simulink model "LR_Traject_Sim"  (R2017b)
settings: Solver=ode4  StartTime=0  StopTime=100  FixedStep=0.05  RelTol=1e-7
model workspace (MAT data in the model file):
  Object = Simulink.LookupTable
  Object.Table = Simulink.lookuptable.Table
  Object.Table.Dimensions = [0 0]
  Object.Table.DataType = 'auto'
  Object.Table.FieldName = 'Table'
  Object.Breakpoints = Simulink.lookuptable.Breakpoint
  Object.Breakpoints.TunableSizeName = 'N1'
  Object.Breakpoints.Dimensions = [0 0]
  Object.Breakpoints.DataType = 'auto'
  Object.Breakpoints.FieldName = 'BP1'
  Object.SupportTunableSize = 0
  Object.StructTypeInfo = Simulink.lookuptable.StructTypeInfo
  Object.StructTypeInfo.DataScope = 'Auto'
values from neighbouring files (symbols this model uses):
  Vull = 0.15    [TestBlowdownModel.m]    (also in runsim.m)
undefined symbols (not defined in the file or in its folder): CEAinterp, Conditions, Eng, Prop, Roc
libraries: simulink x1
settings Model: Creator=adamb  LastModifiedBy=Thomas
settings SolverCC: ZeroCrossAlgorithm=Adaptive
settings DataIOCC: SaveFormat=StructureWithTime
settings OptimizationCC: LifeSpan=inf
settings DebuggingCC: AlgebraicLoopMsg=none  ArtificialAlgebraicLoopMsg=none  SFExecutionAtInitializationDiag=none
settings HardwareCC: ProdBitPerSizeT=32  ProdBitPerPtrDiffT=32  ProdWordSize=32  ProdHWDeviceType=Specified
settings CodeAppCC: StateflowObjectComments=on
settings SimscapeCC: SimscapeNormalizeSystem=off
settings ConfigurationSet: Description=SimMechanics 2G

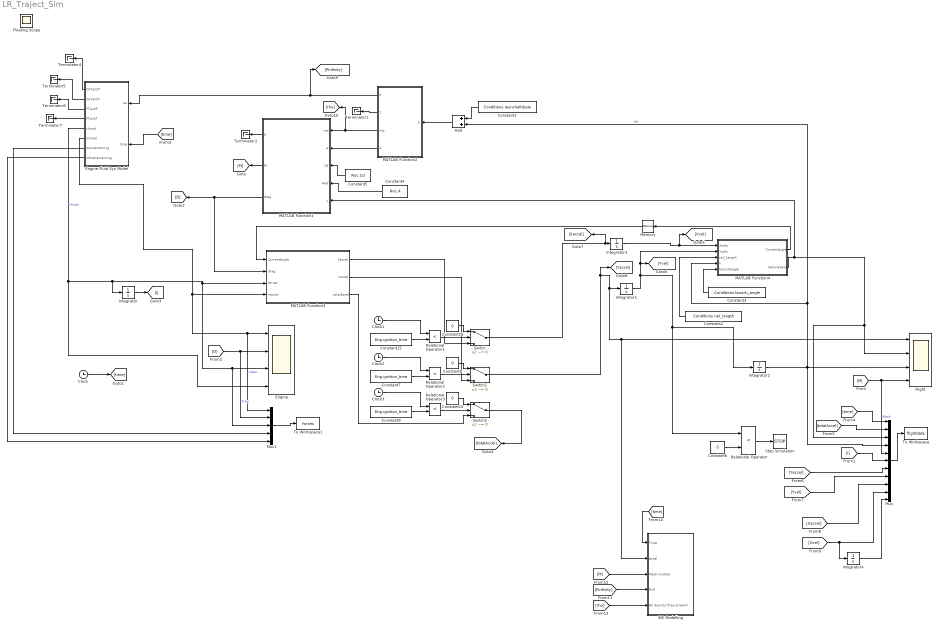
== system LR_Traject_Sim ==
  Add : Sum
  Clock{,1..3} (4 alike) : Clock
  Constant1 : Constant  Value=Conditions.launchaltitude
  Constant10 : Constant  Value=0
  Constant15 : Constant  Value=Eng.ignition_time
  Constant16 : Constant  Value=0
  Constant2 : Constant  Value=Conditions.rail_length
  Constant3 : Constant  Value=Conditions.launch_angle
  Constant4 : Constant  Value=Roc.A
  Constant5 : Constant  Value=Roc.Cd  VectorParams1D=off
  Constant6 : Constant  Value=-5
  Constant7 : Constant  Value=Eng.ignition_time
  Constant8 : Constant  Value=0
  Constant9 : Constant  Value=Eng.ignition_time
  Engine : Scope  NumInputPorts=4
  Engine Fluid Sys Model : Subsystem
  Flight : Scope  NumInputPorts=4
  INS Modelling : Subsystem
  Integrator{,1..4} (5 alike) : Integrator
  MATLAB Function1 : MATLAB Function  TreatAsAtomicUnit=on
  MATLAB Function2 : MATLAB Function  TreatAsAtomicUnit=on
  MATLAB Function3 : MATLAB Function  TreatAsAtomicUnit=on
  MATLAB Function4 : MATLAB Function  TreatAsAtomicUnit=on
  Memory : Memory
  Mux : Mux  Inputs=11
  Mux1 : Mux  Inputs=5
  Relational Operator : RelationalOperator  Operator=<  OutDataTypeStr=boolean  RndMeth=Nearest
  Relational Operator1 : RelationalOperator  Operator=<  OutDataTypeStr=boolean  RndMeth=Simplest
  Relational Operator2 : RelationalOperator  Operator=<  OutDataTypeStr=boolean  RndMeth=Simplest
  Relational Operator3 : RelationalOperator  Operator=<  OutDataTypeStr=boolean  RndMeth=Simplest
  Stop Simulation : Stop
  Switch : Switch  Criteria=u2 ~= 0
  Switch1 : Switch  Criteria=u2 ~= 0
  Switch2 : Switch  Criteria=u2 ~= 0
  Terminator{1..2,4..7} (6 alike) : Terminator
  To Workspace : ToWorkspace  VariableName=flightdata  SampleTime=-1
  To Workspace1 : ToWorkspace  VariableName=forces  SampleTime=-1
  Floating Scope : Scope
  wires:
  Engine Fluid Sys Model/6(mtotal) -> Mux1/1, Engine/1, MATLAB Function3/4(mtotal)  "mass"
  Engine Fluid Sys Model/5(thrust) -> Integrator/1, Mux1/3, Engine/3, MATLAB Function3/3(thrust), Engine/4  "thrust"
  Integrator1/1 -> Relational Operator/1, Integrator2/1, [Yvel], MATLAB Function4/2(Yvelo)
  Integrator2/1 -> Add/2, MATLAB Function4/4(h), Flight/3, Mux/4  "alt"
  Constant4/1 -> MATLAB Function1/4(Aref)
  Constant5/1 -> MATLAB Function1/3(Cd)
  MATLAB Function1/2(M) -> [M]
  [M] -> Mux/5, Flight/4  "Mach"
  MATLAB Function1/3(drag) -> [D], MATLAB Function3/2(drag)
  Relational Operator/1 -> Stop Simulation/1
  Constant6/1 -> Relational Operator/2
  MATLAB Function2/4(a) -> MATLAB Function1/2(a)
  MATLAB Function2/3(rho) -> [rho], MATLAB Function1/1(rho)
  Mux/1 -> To Workspace/1
  MATLAB Function2/2(T) -> Terminator1/1
  [D] -> Mux1/2, Engine/2  "drag"
  Mux1/1 -> To Workspace1/1
  MATLAB Function1/1(q) -> Terminator2/1
  MATLAB Function2/1(P) -> [Pinfinity], Engine Fluid Sys Model/1(pa)
  Clock/1 -> [time]
  [time] -> Engine Fluid Sys Model/2(time)
  [time] -> Mux/1
  Engine Fluid Sys Model/7(moxremaining) -> Mux1/4
  Engine Fluid Sys Model/8(mfuelremaining) -> Mux1/5
  Switch1/1 -> [Yaccel], INS Modelling/2(Accel), Flight/1, Integrator1/1
  Integrator3/1 -> [Xvel], MATLAB Function4/1(Xvelo)
  MATLAB Function4/2(VehicleVelo) -> MATLAB Function1/5(v), Flight/2, Mux/3
  Integrator/1 -> [I]
  [I] -> Mux/6
  Add/1 -> MATLAB Function2/1(h)
  Constant1/1 -> Add/1
  MATLAB Function4/1(CurrentAngle) -> Memory/1
  Engine Fluid Sys Model/1(OxTankP) -> Terminator4/1
  Engine Fluid Sys Model/2(OxTankT) -> Terminator5/1
  Engine Fluid Sys Model/3(FTankP) -> Terminator6/1
  Engine Fluid Sys Model/4(FTankT) -> Terminator7/1
  Constant2/1 -> MATLAB Function4/3(rail_length)
  Constant3/1 -> MATLAB Function4/5(launchangle)
  Memory/1 -> MATLAB Function3/1(CurrentAngle)
  [totalAccel] -> Mux/2
  [Xaccel] -> Mux/9
  [Xvel] -> Integrator4/1, Mux/10
  [Yvel] -> Mux/8
  [Yaccel] -> Mux/7
  Integrator4/1 -> Mux/11
  [time] -> INS Modelling/1(Time)
  [Pinfinity] -> INS Modelling/4(Pinf)
  [M] -> INS Modelling/3(Mach number)
  [rho] -> INS Modelling/5(Air density (free stream))
  Switch/1 -> Integrator3/1, [Xaccel]
  Clock1/1 -> Relational Operator1/1
  Relational Operator1/1 -> Switch/2
  Constant16/1 -> Switch/1
  Constant15/1 -> Relational Operator1/2
  Clock2/1 -> Relational Operator2/1
  Relational Operator2/1 -> Switch1/2
  Constant8/1 -> Switch1/1
  Constant7/1 -> Relational Operator2/2
  Clock3/1 -> Relational Operator3/1
  Relational Operator3/1 -> Switch2/2
  Constant10/1 -> Switch2/1
  Constant9/1 -> Relational Operator3/2
  MATLAB Function3/1(Xaccel) -> Switch/3
  MATLAB Function3/2(Yaccel) -> Switch1/3
  Switch2/1 -> [totalAccel]
  MATLAB Function3/3(totalAccel) -> Switch2/3

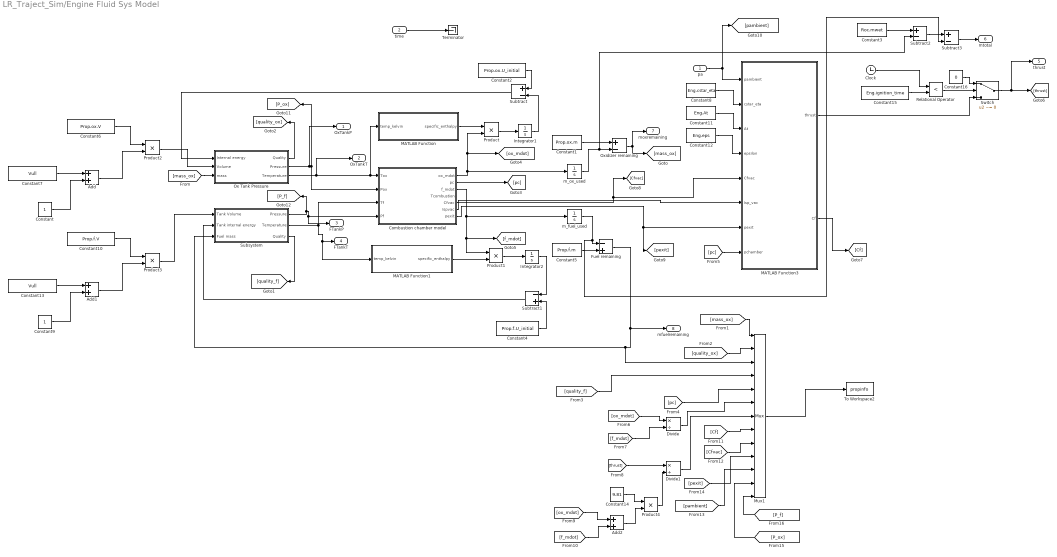
== system LR_Traject_Sim/Engine Fluid Sys Model ==
  pa : Inport
  time : Inport  Port=2
  Add : Sum
  Add1 : Sum
  Add2 : Sum
  Clock : Clock
  Combustion chamber model : Subsystem  TreatAsAtomicUnit=on
  Constant : Constant
  Constant1 : Constant  Value=Prop.ox.m
  Constant10 : Constant  Value=Prop.f.V
  Constant11 : Constant  Value=Eng.At
  Constant12 : Constant  Value=Eng.eps
  Constant13 : Constant  Value=Vull
  Constant14 : Constant  Value=9.81
  Constant15 : Constant  Value=Eng.ignition_time
  Constant16 : Constant  Value=0
  Constant2 : Constant  Value=Prop.ox.U_initial
  Constant3 : Constant  Value=Roc.mwet
  Constant4 : Constant  Value=Prop.f.U_initial
  Constant5 : Constant  Value=Prop.f.m
  Constant6 : Constant  Value=Prop.ox.V
  Constant7 : Constant  Value=Vull
  Constant8 : Constant  Value=Eng.cstar_eta
  Constant9 : Constant
  Divide : Product  Inputs=*/
  Divide1 : Product  Inputs=*/
  Fuel remaining : Sum  Inputs=-+
  Integrator1 : Integrator
  Integrator2 : Integrator
  MATLAB Function : MATLAB Function  TreatAsAtomicUnit=on
  MATLAB Function1 : MATLAB Function  TreatAsAtomicUnit=on
  MATLAB Function3 : MATLAB Function  TreatAsAtomicUnit=on
  Mux1 : Mux  Inputs=13
  Ox Tank Pressure : Subsystem  Variant=on  VariantControl=Variant1
  Oxidizer remaining : Sum  Inputs=+-
  Product{,1..4} (5 alike) : Product
  Relational Operator : RelationalOperator  Operator=<  OutDataTypeStr=boolean  RndMeth=Simplest
  Subsystem : Subsystem
  Subtract : Sum  Inputs=+-
  Subtract1 : Sum  Inputs=-+
  Subtract2 : Sum  Inputs=+-
  Subtract3 : Sum  Inputs=+-
  Switch : Switch  Criteria=u2 ~= 0
  Terminator : Terminator
  To Workspace2 : ToWorkspace  VariableName=propinfo  SampleTime=-1
  m_fuel_used : Integrator
  m_ox_used : Integrator
  OxTankP : Outport
  OxTankT : Outport  Port=2
  FTankP : Outport  Port=3
  FTankT : Outport  Port=4
  thrust : Outport  Port=5
  mtotal : Outport  Port=6
  moxremaining : Outport  Port=7
  mfuelremaining : Outport  Port=8
  wires:
  Constant11/1 -> MATLAB Function3/3(At)
  Constant12/1 -> MATLAB Function3/4(epsilon)
  Constant8/1 -> MATLAB Function3/2(cstar_eta)
  pa/1 -> [pambient], MATLAB Function3/1(pambient)
  Combustion chamber model/1(ox_mdot) -> m_ox_used/1, [ox_mdot], Product/2
  MATLAB Function/1(specific_enthalpy) -> Product/1
  Product/1 -> Integrator1/1
  Integrator1/1 -> Subtract/2
  Product1/1 -> Integrator2/1
  Combustion chamber model/3(f_mdot) -> m_fuel_used/1, [f_mdot], Product1/1
  MATLAB Function1/1(specific_enthalpy) -> Product1/2
  Integrator2/1 -> Subtract1/1
  m_ox_used/1 -> Subtract2/2, Oxidizer remaining/2
  Constant1/1 -> Oxidizer remaining/1
  Oxidizer remaining/1 -> [mass_ox], moxremaining/1
  Constant2/1 -> Subtract/1
  Constant4/1 -> Subtract1/2
  Constant5/1 -> Fuel remaining/2
  m_fuel_used/1 -> Subtract3/2, Fuel remaining/1
  Fuel remaining/1 -> mfuelremaining/1, Subsystem/3(Fuel mass), Mux1/3
  Combustion chamber model/7(pexit) -> [pexit], MATLAB Function3/7(pexit)
  Combustion chamber model/5(Cfvac) -> [Cfvac], MATLAB Function3/5(Cfvac)
  Combustion chamber model/6(Ispvac) -> MATLAB Function3/6(Isp_vac)
  Constant3/1 -> Subtract2/1
  Subtract2/1 -> Subtract3/1
  Subtract3/1 -> mtotal/1
  Constant6/1 -> Product2/1
  Constant7/1 -> Add/1
  Constant/1 -> Add/2
  Add/1 -> Product2/2
  Constant10/1 -> Product3/1
  Constant13/1 -> Add1/1
  Constant9/1 -> Add1/2
  Add1/1 -> Product3/2
  Mux1/1 -> To Workspace2/1
  [mass_ox] -> Mux1/1
  [quality_ox] -> Mux1/2
  [quality_f] -> Mux1/4
  Combustion chamber model/2(pc) -> [pc]
  [pc] -> Mux1/5
  [pc] -> MATLAB Function3/8(pchamber)
  [ox_mdot] -> Divide/1
  [f_mdot] -> Divide/2
  Divide/1 -> Mux1/6
  [ox_mdot] -> Add2/1
  [f_mdot] -> Add2/2
  [thrust] -> Divide1/1
  Product4/1 -> Divide1/2
  Constant14/1 -> Product4/1
  Add2/1 -> Product4/2
  Divide1/1 -> Mux1/7
  MATLAB Function3/2(Cf) -> [Cf]
  [Cf] -> Mux1/8
  [Cfvac] -> Mux1/9
  [pambient] -> Mux1/11
  [pexit] -> Mux1/10
  time/1 -> Terminator/1
  [P_f] -> Mux1/13
  [P_ox] -> Mux1/12
  Subtract/1 -> Ox Tank Pressure/1("Internal energy ")
  Product2/1 -> Ox Tank Pressure/2("Volume ")
  [mass_ox] -> Ox Tank Pressure/3("mass ")
  Ox Tank Pressure/1(" Quality") -> [quality_ox]
  Ox Tank Pressure/2(" Pressure") -> [P_ox], Combustion chamber model/2(Pox), OxTankP/1
  Ox Tank Pressure/3(" Temperature") -> Combustion chamber model/1(Tox), MATLAB Function/1(temp_kelvin), OxTankT/1
  Subsystem/1(Pressure) -> [P_f], FTankP/1, Combustion chamber model/4(Pf)
  Subsystem/2(Temperature) -> MATLAB Function1/1(temp_kelvin), FTankT/1, Combustion chamber model/3(Tf)
  Product3/1 -> Subsystem/1(Tank Volume)
  Subtract1/1 -> Subsystem/2(Tank internal energy)
  Subsystem/3(Quality) -> [quality_f]
  Clock/1 -> Relational Operator/1
  Constant15/1 -> Relational Operator/2
  Relational Operator/1 -> Switch/2
  MATLAB Function3/1(thrust) -> Switch/3
  Constant16/1 -> Switch/1
  Switch/1 -> thrust/1, [thrust]

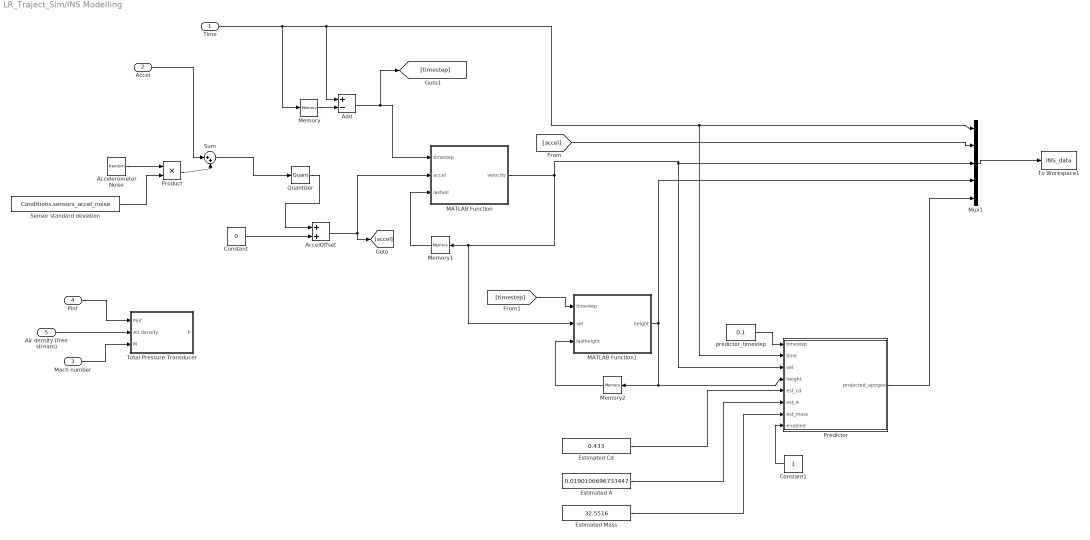
== system LR_Traject_Sim/INS Modelling ==
  Time : Inport  SampleTime=.1
  Accel : Inport  Port=2  SampleTime=.1
  Mach number : Inport  Port=3  SampleTime=.1
  Pinf : Inport  Port=4  SampleTime=.1
  Air density (free stream) : Inport  Port=5  SampleTime=.1
  AccelOffset : Sum
  Accelerometer Noise : RandomNumber  Seed=38778900  SampleTime=0.1  VectorParams1D=off
  Add : Sum  Inputs=+-
  Constant : Constant  Value=0
  Constant1 : Constant
  Estimated A : Constant  Value=0.0190106696733447
  Estimated Cd : Constant  Value=0.433
  Estimated Mass : Constant  Value=32.5516
  MATLAB Function : MATLAB Function  TreatAsAtomicUnit=on
  MATLAB Function1 : MATLAB Function  TreatAsAtomicUnit=on
  Memory : Memory
  Memory1 : Memory
  Memory2 : Memory
  Mux1 : Mux  Inputs=5
  Predictor : MATLAB Function  TreatAsAtomicUnit=on
  Product : Product
  Quantizer : Quantizer  QuantizationInterval=.01
  Sensor standard deviation : Constant  Value=Conditions.sensors_accel_noise
  Sum : Sum  Inputs=|++
  To Workspace1 : ToWorkspace  VariableName=INS_data  SampleTime=.1
  Total Pressure Transducer : Subsystem
  "predictor_timestep " : Constant  Value=0.1
  wires:
  Accel/1 -> Sum/1
  Mux1/1 -> To Workspace1/1
  Time/1 -> Add/1, Predictor/2(time), Mux1/1, Memory/1
  AccelOffset/1 -> MATLAB Function/2(accel), [accel]
  Memory/1 -> Add/2
  Add/1 -> [timestep], MATLAB Function/1(timestep)
  [accel] -> Mux1/2
  MATLAB Function/1(velocity) -> MATLAB Function1/2(vel), Memory1/1, Mux1/3, Predictor/3(vel)
  Memory1/1 -> MATLAB Function/3(lastvel)
  Sum/1 -> Quantizer/1
  [timestep] -> MATLAB Function1/1(timestep)
  MATLAB Function1/1(height) -> Mux1/4, Predictor/4(height), Memory2/1
  Memory2/1 -> MATLAB Function1/3(lastheight)
  Predictor/1(projected_apogee) -> Mux1/5
  Quantizer/1 -> AccelOffset/1
  Constant/1 -> AccelOffset/2
  Estimated Cd/1 -> Predictor/5(est_cd)
  Estimated A/1 -> Predictor/6(est_A)
  Estimated Mass/1 -> Predictor/7(est_mass)
  "predictor_timestep "/1 -> Predictor/1(timestep)
  Sensor standard deviation/1 -> Product/2
  Accelerometer Noise/1 -> Product/1
  Product/1 -> Sum/2
  Constant1/1 -> Predictor/8(enabled)
  Pinf/1 -> Total Pressure Transducer/1(Pinf)
  Mach number/1 -> Total Pressure Transducer/3(M)
  Air density (free stream)/1 -> Total Pressure Transducer/2(Air density)

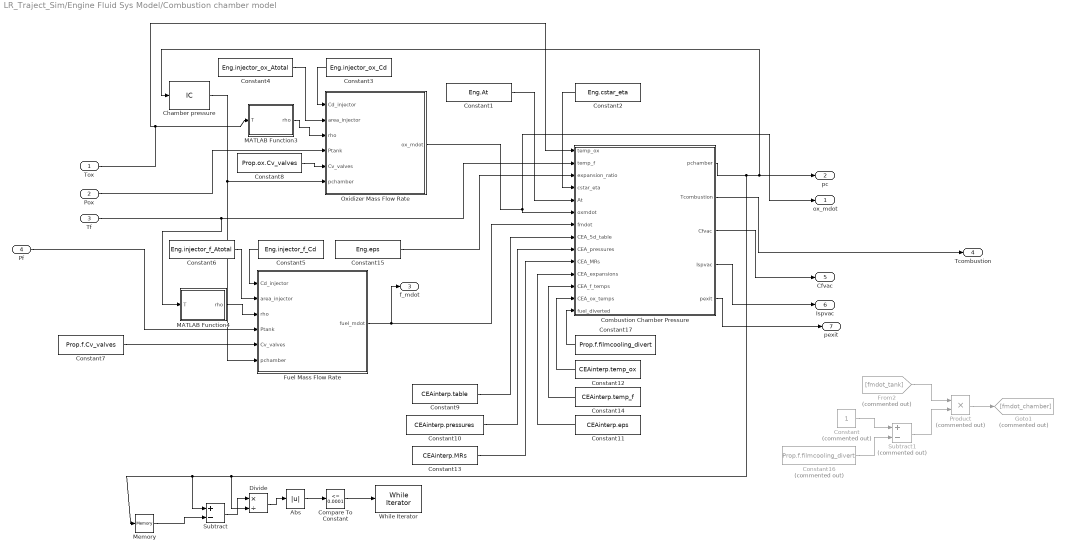
== system LR_Traject_Sim/Engine Fluid Sys Model/Combustion chamber model ==
  Tox : Inport
  Pox : Inport  Port=2
  Tf : Inport  Port=3
  Pf : Inport  Port=4
  Abs : Abs
  "Chamber pressure " : InitialCondition  Value=2000000
  Combustion Chamber Pressure : MATLAB Function
      settings: MinAlgLoopOccurrences=on
  Compare To Constant : simulink/Logic and Bit Operations/Compare To Constant  relop=<=  const=0.0001  OutDataTypeStr=boolean
  Constant : Constant  Commented=on
  Constant1 : Constant  Value=Eng.At
  Constant10 : Constant  Value=CEAinterp.pressures
  Constant11 : Constant  Value=CEAinterp.eps
  Constant12 : Constant  Value=CEAinterp.temp_ox
  Constant13 : Constant  Value=CEAinterp.MRs
  Constant14 : Constant  Value=CEAinterp.temp_f
  Constant15 : Constant  Value=Eng.eps
  Constant16 : Constant  Commented=on  Value=Prop.f.filmcooling_divert
  Constant17 : Constant  Value=Prop.f.filmcooling_divert
  Constant2 : Constant  Value=Eng.cstar_eta
  Constant3 : Constant  Value=Eng.injector_ox_Cd
  Constant4 : Constant  Value=Eng.injector_ox_Atotal
  Constant5 : Constant  Value=Eng.injector_f_Cd
  Constant6 : Constant  Value=Eng.injector_f_Atotal
  Constant7 : Constant  Value=Prop.f.Cv_valves
  Constant8 : Constant  Value=Prop.ox.Cv_valves
  Constant9 : Constant  Value=CEAinterp.table
  Divide : Product  Inputs=*/
  From2 : From  Commented=on  GotoTag=fmdot_tank
  Fuel Mass Flow Rate : MATLAB Function
      settings: MinAlgLoopOccurrences=on
  Goto1 : Goto  Commented=on  GotoTag=fmdot_chamber
  MATLAB Function3 : MATLAB Function
      settings: MinAlgLoopOccurrences=on
  MATLAB Function4 : MATLAB Function
      settings: MinAlgLoopOccurrences=on
  Memory : Memory  InheritSampleTime=on
  Oxidizer Mass Flow Rate : MATLAB Function
      settings: MinAlgLoopOccurrences=on
  Product : Product  Commented=on
  Subtract : Sum  Inputs=+-
  Subtract1 : Sum  Commented=on  Inputs=+-
  While Iterator : WhileIterator  MaxIters=50  WhileBlockType=do-while
  ox_mdot : Outport
  pc : Outport  Port=2
  f_mdot : Outport  Port=3
  Tcombustion : Outport  Port=4
  Cfvac : Outport  Port=5
  Ispvac : Outport  Port=6
  pexit : Outport  Port=7
  wires:
  Oxidizer Mass Flow Rate/1(ox_mdot) -> ox_mdot/1, Combustion Chamber Pressure/6(oxmdot)
  Constant13/1 -> Combustion Chamber Pressure/10(CEA_MRs)
  Constant9/1 -> Combustion Chamber Pressure/8(CEA_5d_table)
  Constant10/1 -> Combustion Chamber Pressure/9(CEA_pressures)
  Pox/1 -> Oxidizer Mass Flow Rate/4(Ptank)
  Pf/1 -> Fuel Mass Flow Rate/4(Ptank)
  Combustion Chamber Pressure/1(pchamber) -> Divide/2, Subtract/1, Memory/1, "Chamber pressure "/1, pc/1
  Memory/1 -> Subtract/2
  Subtract/1 -> Divide/1
  Divide/1 -> Abs/1
  Abs/1 -> Compare To Constant/1
  Compare To Constant/1 -> While Iterator/1
  Combustion Chamber Pressure/5(pexit) -> pexit/1
  "Chamber pressure "/1 -> Oxidizer Mass Flow Rate/6(pchamber), Fuel Mass Flow Rate/6(pchamber)
  Constant1/1 -> Combustion Chamber Pressure/5(At)
  Constant2/1 -> Combustion Chamber Pressure/4(cstar_eta)
  Constant3/1 -> Oxidizer Mass Flow Rate/1(Cd_injector)
  Constant4/1 -> Oxidizer Mass Flow Rate/2(area_injector)
  MATLAB Function3/1(rho) -> Oxidizer Mass Flow Rate/3(rho)
  Tox/1 -> MATLAB Function3/1(T), Combustion Chamber Pressure/1(temp_ox)
  MATLAB Function4/1(rho) -> Fuel Mass Flow Rate/3(rho)
  Tf/1 -> Combustion Chamber Pressure/2(temp_f), MATLAB Function4/1(T)
  Constant5/1 -> Fuel Mass Flow Rate/1(Cd_injector)
  Constant6/1 -> Fuel Mass Flow Rate/2(area_injector)
  Constant7/1 -> Fuel Mass Flow Rate/5(Cv_valves)
  Constant8/1 -> Oxidizer Mass Flow Rate/5(Cv_valves)
  Constant12/1 -> Combustion Chamber Pressure/13(CEA_ox_temps)
  Constant14/1 -> Combustion Chamber Pressure/12(CEA_f_temps)
  Constant11/1 -> Combustion Chamber Pressure/11(CEA_expansions)
  Constant15/1 -> Combustion Chamber Pressure/3(expansion_ratio)
  Combustion Chamber Pressure/2(Tcombustion) -> Tcombustion/1
  Combustion Chamber Pressure/3(Cfvac) -> Cfvac/1
  Combustion Chamber Pressure/4(Ispvac) -> Ispvac/1
  Constant/1 -> Subtract1/1
  Constant16/1 -> Subtract1/2
  From2/1 -> Product/1
  Subtract1/1 -> Product/2
  Product/1 -> Goto1/1
  Fuel Mass Flow Rate/1(fuel_mdot) -> Combustion Chamber Pressure/7(fmdot), f_mdot/1
  Constant17/1 -> Combustion Chamber Pressure/14(fuel_diverted)

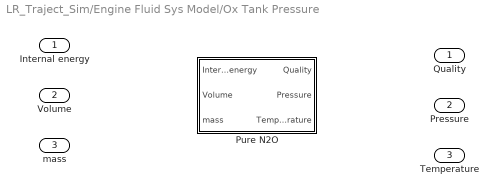
== system LR_Traject_Sim/Engine Fluid Sys Model/Ox Tank Pressure ==
  "Internal energy " : Inport
  "Volume " : Inport  Port=2
  "mass " : Inport  Port=3
  Pure N2O : Subsystem  VariantControl=PureNitrous
  " Quality" : Outport
  " Pressure" : Outport  Port=2
  " Temperature" : Outport  Port=3

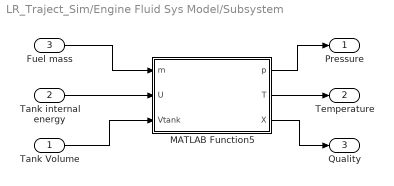
== system LR_Traject_Sim/Engine Fluid Sys Model/Subsystem ==
  Tank Volume : Inport
  Tank internal energy : Inport  Port=2
  Fuel mass : Inport  Port=3
  MATLAB Function5 : MATLAB Function  TreatAsAtomicUnit=on
  Pressure : Outport
  Temperature : Outport  Port=2
  Quality : Outport  Port=3
  wires:
  MATLAB Function5/1(p) -> Pressure/1
  MATLAB Function5/2(T) -> Temperature/1
  Tank internal energy/1 -> MATLAB Function5/2(U)
  MATLAB Function5/3(X) -> Quality/1
  Tank Volume/1 -> MATLAB Function5/3(Vtank)
  Fuel mass/1 -> MATLAB Function5/1(m)

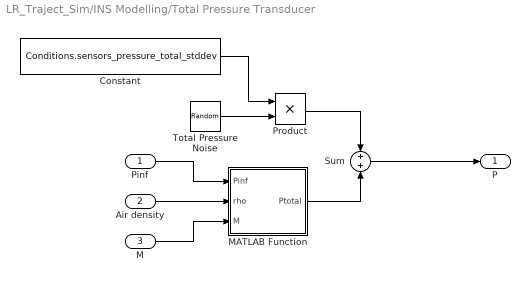
== system LR_Traject_Sim/INS Modelling/Total Pressure Transducer ==
  Pinf : Inport
  Air density : Inport  Port=2
  M : Inport  Port=3
  Constant : Constant  Value=Conditions.sensors_pressure_total_stddev
  MATLAB Function : MATLAB Function  TreatAsAtomicUnit=on
  Product : Product
  Sum : Sum
  Total Pressure Noise : RandomNumber  Seed=23534700  SampleTime=0.1  VectorParams1D=off
  P : Outport
  wires:
  M/1 -> MATLAB Function/3(M)
  Pinf/1 -> MATLAB Function/1(Pinf)
  MATLAB Function/1(Ptotal) -> Sum/2
  Sum/1 -> P/1
  Product/1 -> Sum/1
  Total Pressure Noise/1 -> Product/2
  Constant/1 -> Product/1
  Air density/1 -> MATLAB Function/2(rho)

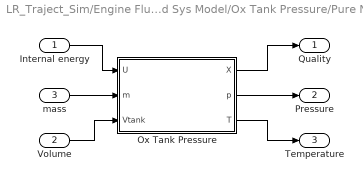
== system LR_Traject_Sim/Engine Fluid Sys Model/Ox Tank Pressure/Pure N2O ==
  "Internal energy " : Inport
  "Volume " : Inport  Port=2
  "mass " : Inport  Port=3
  Ox Tank Pressure : MATLAB Function  TreatAsAtomicUnit=on
  " Quality" : Outport
  " Pressure" : Outport  Port=2
  " Temperature" : Outport  Port=3
  wires:
  Ox Tank Pressure/2(p) -> " Pressure"/1
  Ox Tank Pressure/3(T) -> " Temperature"/1
  "Internal energy "/1 -> Ox Tank Pressure/1(U)
  "Volume "/1 -> Ox Tank Pressure/3(Vtank)
  Ox Tank Pressure/1(X) -> " Quality"/1
  "mass "/1 -> Ox Tank Pressure/2(m)

== matlab function LR_Traject_Sim/MATLAB Function1 ==
  data: rho input; a input; q output; M output; Cd input; Aref input; v input; drag output
function [q,M,drag] = AeroComputation(rho,a,Cd,Aref,v)

M = abs(v/a); % Mach #
q = 0.5*rho*abs(v)*v; % qbar, Dynamic Pressure

A = Aref(1);
CdM = interp1(Cd(1,:),Cd(2,:),M); % Interpolates the Cd based on M

drag = q*A*CdM;

%fprintf('Velocity is %f, drag is %f, rho is %f, a is %f, Cdm is %f\n', v, drag, rho, a, CdM);


end

== matlab function LR_Traject_Sim/INS Modelling/MATLAB Function ==
  data: timestep input; accel input; lastvel input; velocity output
function velocity = fcn(timestep, accel, lastvel)
velocity = lastvel + timestep * accel;
end

== matlab function LR_Traject_Sim/MATLAB Function2 ==
  data: h input; P output; T output; rho output; a output
function [P,T,rho,a] = AtmosParams(h)

[P,rho,T,a] = StdAtmos(h);

end

== matlab function LR_Traject_Sim/Engine Fluid Sys Model/MATLAB Function3 ==
  data: pambient input; cstar_eta input; At input; thrust output; epsilon input; Cfvac input; Isp_vac input; pexit input; pchamber input; Cf output
function [thrust, Cf] = ThrustCalc(pambient, cstar_eta, At, epsilon, Cfvac, Isp_vac, pexit, pchamber)

psitoPa = 6894.76; % [Pa/psi]
maxIt = 400;
conv_crit = 0.001;
g = 9.81; % [m/s^2]
% Determine chamber pressure
if pchamber == 0
    thrust = 0;
    Cf = 0;
    return;
end

%Tc = data(1); % Chamber Temperature (try to keep it low)
%Cfvac = data(2); % Exit thrust coefficient, vacuum
%Isp_vac = data(3); % Vacuum Isp [s]
cstar_th = (g * Isp_vac) / Cfvac; % Theoretical C* [m/s]
cstar = cstar_th * cstar_eta; % Expected C* at efficiency determined [m/s]
pe = pexit; %data(4); % Exit Pressure [Pa]
Cfp = eps * ((pe - pambient) / pchamber); % Pressure term thrust coefficient
Cf = Cfvac + Cfp; % Actual thrust coefficient

% Actual thrust coefficient 
Cf = Cfvac + (epsilon * At) * ((pe - pambient) / pchamber);
% Output thrust
thrust = pchamber * At * Cf; % [N]

%fprintf('Thrust is %f\n', thrust);

end

function ret = CEA_interp(table, pressures, MRs, p, mr)
coder.extrinsic('warning');
ret = [5 5 5 5];
if p < min(pressures) || p > max(pressures)
    fprintf('p is %f\n', p);
    fprintf('min press is %f, max press is %f\n', min(pressures), max(pressures));
    warning('Sample pressure outside interpolation range');
%     slope = (table(end, :, :) - table(end - 1, :, :)) / (pressures(end) - pressures(end - 1));
%     newrow = 
end

if mr < min(MRs) || mr > max(MRs)
    warning('Sample mixture ratio outside interpolation range');
end

for r = 1:length(pressures)
    if p >= pressures(r) && p <= pressures(r + 1)
    	for c = 1:length(MRs)
            if mr >= MRs(c) && mr <= MRs(c + 1)
                pfrac = (p - pressures(r)) / (pressures(r + 1) - pressures(r));
                cfrac = (mr - MRs(r)) / (MRs(r + 1) - MRs(r));
                
                c1 = table(r, c, :) + pfrac * (table(r + 1, c, :) - table(r, c, :));
                c2 = table(r, c + 1, :) + pfrac * (table(r + 1, c + 1, :) - table(r, c + 1, :));
                ret = c1 + cfrac * (c2 - c1);
                break;
            end
        end
        break;
    end
end
end

== matlab function LR_Traject_Sim/Engine Fluid Sys Model/Ox Tank Pressure/Pure N2O/Ox Tank Pressure ==
  data: X output; U input; p output; T output; m input; Vtank input
function [X, p, T] = oxtankpressure(U, m, Vtank)
% Oxygen tank pressure, temperature, and mass flow rate
% psitoPa = 6894.76; % [Pa/psi]
% 
% p_psi = 300;
% 
% p = 4.182e+06; %p_psi * psitoPa;
% mdot = 1.0; % [kg/s]
% T = 285; % [K]
% if m <= 0
%     p = 0;
% end
iter = 0;
Ti = 295;
ET = 0;
T = 300;
xi = 0.5;
err = 0; % Need to define it out of the scope of the loop to use below
while iter < 75
%     ul = liquid_u(Ti);
%     uv = vapor_u(Ti);
%     xi = (U/m - ul)/(uv-ul);
%     rhol = liquid_rho(Ti);
%     rhov = vapor_rho(Ti);
%     mchk = Vtank * ((1-xi)/rhol + xi/rhov)^(-1);
    [mchk, xi] = get_tank_mass(Ti, m, Vtank, U);
    dmdT = (get_tank_mass(Ti + 1, m, Vtank, U) - get_tank_mass(Ti - 1, m, Vtank, U)) / 2;
    
    ETi = m - mchk;
    dE = (ETi - ET)/(Ti-T);
    Tnew = Ti + (m - mchk)/dmdT;
    if Tnew > 309
        Tnew = 309;
    end
    %err = (Tnew - Ti)/Tnew; % This one is crappy 
    err = ETi/m;
    if abs(err) < 0.00005
        break
    end
    ET = ETi;
    T = Ti;
    Ti = Tnew;
    iter = iter+1;
end

p = pressure_eq(T);

if xi >= 1
%     propFlag = 0; % No more liquid
    xi = 1;
    p = 0;
end
%fprintf('P is %f, T is %f\n', p, T);

X = xi;

end

function [m, x] = get_tank_mass(T, m, Vtank, U)
ul = liquid_u(T);
uv = vapor_u(T);
x = (U/m - ul)/(uv-ul);
rhol = liquid_rho(T);
rhov = vapor_rho(T);
m = Vtank * ((1-x)/rhol + x/rhov)^(-1);
end

function u = vapor_u(T)
Trange = 260:1:309;
res = [362468.410284606,362489.391123008,362497.729905660,362493.013314485,362474.805635817,362442.646977473,362396.051299488,362334.504234311,362257.460668461,362164.342053176,362054.533406200,361927.379960487,361782.183407995,361618.197677396,361434.624173463,361230.606392224,361005.223809364,360757.484918858,360486.319273493,360190.568347412,359868.975001232,359520.171280432,359142.664214230,358734.819200865,358294.840460090,357820.747896595,357310.349537569,356761.208467350,356170.602858767,355535.477260287,354852.382689927,354117.402235156,353326.057646064,352473.190654482,351552.810162316,350557.892538843,349480.116240655,348309.502413277,347033.917518239,345638.367609418,344103.967355847,342406.381042271,340513.365243914,338380.693231274,335944.948065437,333109.670491083,329715.531955556,325464.533816668,319667.143315152,309719.712616756];
u = interp1(Trange, res, T);
end

function u = liquid_u(T)
Trange = 260:1:309;
res = [135446.500036654,137417.933720485,139397.647568132,141385.915892570,143383.027874483,145389.288799296,147405.021425607,149430.567502331,151466.289454597,153512.572261677,155569.825554133,157638.485961985,159719.019751281,161811.925793193,163917.738917931,166037.033715727,168170.428859347,170318.592037666,172482.245608510,174662.173102236,176859.226736877,179074.336142620,181308.518540671,183562.890682181,185838.682931504,188137.255980873,190460.120819297,192808.962759647,195185.670572433,197592.372108916,200031.478258993,202505.737739569,205018.306137641,207572.833981365,210173.580610954,212825.563645980,215534.758535051,218308.370142405,221155.210590880,224086.238439105,227115.351208857,230260.591863263,233546.064549798,237005.138156628,240686.164089424,244663.584898171,249062.161783212,254119.534584400,260399.478111094,270124.473783683];
u = interp1(Trange, res, T);
end

function r = vapor_rho(T)
Trange = 260:1:309;
res = [57.5794861418367,59.3387058711366,61.1467347808766,63.0051923645867,64.9157859114953,66.8803175860175,68.9006922492387,70.9789261193159,73.1171563829797,75.3176518884480,77.5828250715845,79.9152452930464,82.3176537948797,84.7929805226673,87.3443631043623,89.9751683321873,92.6890165614642,95.4898095233951,98.3817621517996,101.369439152191,104.457797202683,107.652233879728,110.958644660887,114.383489689313,117.933872415100,121.617632790723,125.443458439242,129.421018202110,133.561123805548,137.875927202369,142.379163660433,147.086454196972,152.015685988187,157.187496681464,162.625899332024,168.359100997349,174.420593268207,180.850633152444,187.698298517684,195.024413963668,202.905840316772,211.441986464954,220.765118372611,231.057541463456,242.582155556968,255.741567820138,271.206370509851,290.244294979758,315.832472913960,359.499534584565];
r = interp1(Trange, res, T);
end

function r = liquid_rho(T)
Trange = 260:1:309;
res = [968.960538442119,964.555134684085,960.106382836984,955.612841552275,951.072988141343,946.485211815440,941.847806201344,937.158961037201,932.416752937820,927.619135100764,922.763925803109,917.848795513144,912.871252410477,907.828626070798,902.718049026446,897.536435858909,892.280459411956,886.946523630991,881.530732431160,876.028853868183,870.436278724405,864.747972418334,858.958418885733,853.061554746050,847.050691635084,840.918424018788,834.656519056104,828.255784082237,821.705905939430,814.995254546292,808.110640555655,801.037013382711,793.757080794342,786.250823859861,778.494870124842,770.461671330684,762.118406390499,753.425489589513,744.334497162176,734.785211936459,724.701285144904,713.983642756544,702.500035071622,690.067600177291,676.421826448870,661.156451382789,643.592930453763,622.445242940298,594.686390337048,548.570585740960];
r = interp1(Trange, res, T);
end

function p = pressure_eq(T)
Trange = 260:1:309;
res = [2192043.44930278,2254565.22513403,2318374.50169227,2383487.73254715,2449921.53375974,2517692.69383879,2586818.18453088,2657315.17252395,2729201.03215190,2802493.35919912,2877209.98591676,2953368.99737765,3030988.74931267,3110087.88759292,3190685.36954337,3272800.48730302,3356452.89347669,3441662.62936488,3528450.15609900,3616836.38906907,3706842.73609295,3798491.13985669,3891804.12525400,3986804.85236920,4083517.17599827,4181965.71278260,4282175.91726328,4384174.16845224,4487987.86889146,4593645.55865130,4701177.04734807,4810613.56809249,4921987.95839212,5035334.87454610,5150691.04815519,5268095.59630831,5387590.40120857,5509220.58116494,5633035.08412362,5759087.44920981,5887436.80456204,6018149.20757225,6151299.49924542,6286973.96447160,6425274.32483282,6566324.08985303,6710279.47689546,6857350.37801454,7007848.18845096,7162336.96521168];
p = interp1(Trange, res, T);
end

== matlab function LR_Traject_Sim/Engine Fluid Sys Model/Subsystem/MATLAB Function5 ==
  data: m input; U input; p output; T output; Vtank input; X output
function [p, T, X] = fueltankpressure(m, U, Vtank)
% Oxygen tank pressure, temperature, and mass flow rate
iter = 0;
Ti = 295;
ET = 0;
T = 300;
xi = 0.5;
while iter < 75
%     ul = liquid_u(Ti);
%     uv = vapor_u(Ti);
%     xi = (U/m - ul)/(uv-ul);
%     rhol = liquid_rho(Ti);
%     rhov = vapor_rho(Ti);
%     mchk = Vtank * ((1-xi)/rhol + xi/rhov)^(-1);
    
    [mchk, xi] = get_tank_mass(Ti, m, Vtank, U);
    dmdT = (get_tank_mass(Ti + 1, m, Vtank, U) - get_tank_mass(Ti - 1, m, Vtank, U)) / 2;
    
    ETi = m - mchk;
    dE = (ETi - ET)/(Ti-T);
    Tnew = Ti + (m - mchk)/dmdT;
    %fprintf('dmdT = %f, Tnew = %f\n', dmdT, Tnew);
    if Tnew > 305
        Tnew = 305;
    end
    %err = (Tnew - Ti)/Tnew; % This one is crappy 
    err = ETi/m;
    if abs(err) < 0.00005
        break
    end
    ET = ETi;
    T = Ti;
    Ti = Tnew;
    iter = iter+1;
end

p = pressure_eq(T);
if xi >= 1
%     propFlag = 0; % No more liquid
    xi = 1;
    p = 0;
end
%fprintf('P is %f, T is %f\n', p, T);
%fprintf('T = %f, P = %f\n', T, p);
X = xi;

end

function [m, x] = get_tank_mass(T, m, Vtank, U)
ul = liquid_u(T);
uv = vapor_u(T);
x = (U/m - ul)/(uv-ul);
rhol = liquid_rho(T);
rhov = vapor_rho(T);
m = Vtank * ((1-x)/rhol + x/rhov)^(-1);
end

function u = vapor_u(T)
Trange = 260:1:305;
res = [496032.650046679,496407.073062043,496762.613644506,497098.523390139,497414.008177858,497708.224552580,497980.275750465,498229.207284278,498454.001989207,498653.574411482,498826.764403699,498972.329771366,499088.937794021,499175.155419687,499229.437901481,499250.115607253,499235.378683815,499183.259192611,499091.610248207,498958.081578202,498780.090774065,498554.789305099,498279.022105509,497949.279193996,497561.637312422,497111.688925618,496594.455034507,496004.277008482,495334.680869123,494578.204887583,493726.177561557,492768.427306705,491692.896335470,490485.117118734,489127.486770510,487598.235597782,485869.917022481,483907.118280360,481662.840975006,479072.475449476,476043.093121210,472432.720550894,468005.203218850,462313.034786665,454286.510541325,439176.751505796];
u = interp1(Trange, res, T);
end

function u = liquid_u(T)
Trange = 260:1:305;
res = [200890.750662334,203934.947987449,206995.976307644,210074.367322168,213170.683421954,216285.520421680,219419.510599113,222573.326091328,225747.682675511,228943.343994826,232161.126287818,235401.903698654,238666.614264649,241956.266702582,245271.948147222,248614.833035226,251986.193376898,255387.410719274,258819.990179360,262285.577020158,265785.976359792,269323.176753606,272899.378581596,276517.028425416,280178.860953497,283887.950284329,287647.773417551,291462.289187995,295336.037429132,299274.264818752,303283.086526962,307369.696800964,311542.647864077,315812.226489841,320190.974081529,324694.424229098,329342.181780979,334159.560824368,339180.183058485,344450.326603351,350036.708186694,356041.672121498,362636.580179410,370149.435701877,379376.697787779,393981.950893429];
u = interp1(Trange, res, T);
end

function r = vapor_rho(T)
Trange = 260:1:305;
res = [31.5784493144864,32.5012353936404,33.4497295206374,34.4248705575019,35.4276544660015,36.4591393119683,37.5204508378625,38.6127886869962,39.7374333778250,40.8957541446636,42.0892177827159,43.3193986613596,44.5879901012861,45.8968173499029,47.2478524373221,48.6432312548466,50.0852732725996,51.5765044073408,53.1196836717464,54.7178343907895,56.3742809707655,58.0926924677305,59.8771345468333,61.7321318836698,63.6627436787100,65.6746558022495,67.7742942585768,69.9689663026843,72.2670378894365,74.6781595428242,77.2135577785265,79.8864168466907,82.7123873923134,85.7102774681517,88.9030122643567,92.3190015158986,95.9941467018075,99.9748931810239,104.323072584020,109.123997304899,114.500913588321,120.643136271340,127.867738638966,136.781049110291,148.851266462714,170.754818367359];
r = interp1(Trange, res, T);
end

function r = liquid_rho(T)
Trange = 260:1:305;
res = [429.076168213018,427.062467606728,425.024398601393,422.961031163630,420.871379098400,418.754395003084,416.608964568072,414.433900112595,412.227933273765,409.989706722213,407.717764782997,405.410542818095,403.066355204805,400.683381713451,398.259652045502,395.793028236011,393.281184547713,390.721584382754,388.111453605412,385.447749496481,382.727124336404,379.945882324264,377.099928162542,374.184705142865,371.195119912639,368.125450222587,364.969230755463,361.719110472184,358.366672559390,354.902204669442,351.314402140713,347.589979331509,343.713152495257,339.664938963627,335.422186701185,330.956195950623,326.230701746571,321.198813070513,315.798163820590,309.942813058736,303.508785779834,296.305932390545,288.016278700313,278.032969408980,264.891193367290,241.961491087650];
r = interp1(Trange, res, T);
end

function p = pressure_eq(T)
Trange = 260:1:305;
res = [1711835.43806923,1757550.88035733,1804147.62260265,1851636.51600566,1900028.54094022,1949334.81436071,1999566.59852213,2050735.30921139,2102852.52572953,2155930.00130072,2209979.67452346,2265013.68191541,2321044.37169553,2378084.31896794,2436146.34249589,2495243.52327889,2555389.22517910,2616597.11787405,2678881.20245765,2742255.84005632,2806735.78388548,2872336.21524109,2939072.78400749,3006961.65437044,3076019.55656555,3146263.84567555,3217712.56873433,3290384.54173006,3364299.43855660,3439477.89460487,3515941.62859555,3593713.58756242,3672818.12180763,3753281.19948600,3835130.67476294,3918396.63011162,4003111.82380483,4089312.29081872,4177038.17458039,4266334.91936507,4357255.05358123,4449861.00495574,4544229.88931892,4640462.63613746,4738705.16050522,4839225.04388939];
p = interp1(Trange, res, T);
end

== matlab function LR_Traject_Sim/Engine Fluid Sys Model/Combustion chamber model/Oxidizer Mass Flow Rate ==
  data: Cd_injector input; ox_mdot output; area_injector input; rho input; Ptank input; Cv_valves input; pchamber input
function ox_mdot = ox_mdot_calculation(Cd_injector, area_injector, rho, Ptank, Cv_valves, pchamber)

rho_h2o = 998; %kg/m^3
mdot_guess = 1; % kg/s
%error = @(mdot) mdot - Cd_injector * area_injector * sqrt(2 * rho * (Ptank - mdot^2 / (Cv_valves^2 * rho * roe_h2o) - pchamber));
%ox_mdot = fzero(error, mdot_guess);
if Ptank == 0
    ox_mdot = 0;
    return;
end
min = 0.01; % [kg/s]
max = 3; % [kg/s]
res = 1;
maxIt = 200;
for n = 1:maxIt
    avg = (min + max) / 2;
    res = error(avg, Cd_injector, area_injector, rho, Ptank, Cv_valves, pchamber, rho_h2o);
    if abs((avg-res) / res) < 0.0001
        break;
    end
    if res > avg
        max = avg;
    else
        min = avg;
    end
end
ox_mdot = res;

end

function md = error(mdot, Cd_injector, area_injector, rho, Ptank, Cv_valves, pchamber, rho_h2o)
md = Cd_injector * area_injector * sqrt(2 * rho * (Ptank - mdot^2 / (Cv_valves^2 * rho * rho_h2o) - pchamber));
end

== matlab function LR_Traject_Sim/Engine Fluid Sys Model/Combustion chamber model/Combustion Chamber Pressure ==
  data: temp_ox input; temp_f input; expansion_ratio input; pchamber output; Tcombustion output; Cfvac output; Ispvac output; cstar_eta input; At input; oxmdot input; fmdot input; CEA_5d_table input; CEA_pressures input; CEA_MRs input; pexit output; CEA_expansions input; CEA_f_temps input; CEA_ox_temps input; fuel_diverted input
function [pchamber, Tcombustion, Cfvac, Ispvac, pexit] = chamberpressurecalc(temp_ox, temp_f, expansion_ratio, cstar_eta, At, oxmdot, fmdot, CEA_5d_table, CEA_pressures, CEA_MRs, CEA_expansions, CEA_f_temps, CEA_ox_temps, fuel_diverted)
fmdot = fmdot * (1 - fuel_diverted);
psitoPa = 6894.76; % [Pa/psi]
maxIt = 400;
conv_crit = 0.001;
% Determine chamber pressure
%fprintf('Fmdot is %f\n', fmdot);
if fmdot == 0 || oxmdot == 0
    pchamber = 0;
    Tcombustion = 0;
    Cfvac = 0;
    Ispvac = 0;
    pexit = 0;
    return;
end

%Iteration begin
pchamber = 300 * psitoPa; % Initial guess [Pa]
g = 9.81; % m/s^2
for n = 1:maxIt
    %[data] = CEA_Rocket(char(Prop.ox.name(2)),char(Prop.f.name(2)), pchamber, oxmdot / fmdot, epsilon, Tamb, Tamb);
%     fprintf('Pchamber was %f\n', pchamber);
    [data] = scatter_5d_interp(CEA_pressures, CEA_MRs, CEA_expansions, CEA_ox_temps, CEA_f_temps, CEA_5d_table, [pchamber, oxmdot / fmdot, expansion_ratio, temp_ox, temp_f]);
%     fprintf('Data is %f, %f, %f, %f\n', data(1), data(2), data(3), data(4));
    Cfvac = data(2); % Exit thrust coefficient, vacuum
    Isp_vac = data(3); % Vacuum Isp [s]
    cstar_th = (g * Isp_vac) / Cfvac; % Theoretical C* [m/s]
    cstar = cstar_th * cstar_eta; % Expected C* at efficiency determined [m/s]
    
    pnew = cstar * (oxmdot + fmdot) / At;
    
    Tcombustion = data(1);
    Cfvac = data(2);
    Ispvac = data(3);
    pexit = data(4);
    
    if abs((pnew - pchamber) / pnew) < conv_crit
        pchamber = pnew;
        break;
    else
        pchamber = pnew;
    end
end
end

function ret = CEA_interp(table, pressures, MRs, p, mr)
coder.extrinsic('warning');
ret = [5 5 5 5];
if p < min(pressures) || p > max(pressures)
    fprintf('p is %f\n', p);
    fprintf('min press is %f, max press is %f\n', min(pressures), max(pressures));
    warning('Sample pressure outside interpolation range');
%     slope = (table(end, :, :) - table(end - 1, :, :)) / (pressures(end) - pressures(end - 1));
%     newrow = 
end

if mr < min(MRs) || mr > max(MRs)
    warning('Sample mixture ratio outside interpolation range');
end

for r = 1:length(pressures)
    if p >= pressures(r) && p <= pressures(r + 1)
    	for c = 1:length(MRs)
            if mr >= MRs(c) && mr <= MRs(c + 1)
                pfrac = (p - pressures(r)) / (pressures(r + 1) - pressures(r));
                cfrac = (mr - MRs(r)) / (MRs(r + 1) - MRs(r));
                
                c1 = table(r, c, :) + pfrac * (table(r + 1, c, :) - table(r, c, :));
                c2 = table(r, c + 1, :) + pfrac * (table(r + 1, c + 1, :) - table(r, c + 1, :));
                ret = c1 + cfrac * (c2 - c1);
                break;
            end
        end
        break;
    end
end
end

== matlab function LR_Traject_Sim/Engine Fluid Sys Model/Combustion chamber model/Fuel Mass Flow Rate ==
  data: Cd_injector input; fuel_mdot output; area_injector input; rho input; Ptank input; Cv_valves input; pchamber input
function fuel_mdot = fuel_mdot_calculation(Cd_injector, area_injector, rho, Ptank, Cv_valves, pchamber)

rho_h2o = 998; %kg/m^3
mdot_guess = 1; % kg/s
%error = @(mdot) mdot - Cd_injector * area_injector * sqrt(2 * rho * (Ptank - mdot^2 / (Cv_valves^2 * rho * roe_h2o) - pchamber));

if Ptank == 0
    fuel_mdot = 0;
    return;
end
%fuel_mdot = fzero(error, mdot_guess);
min = 0.01; % [kg/s]
max = 3; % [kg/s]
res = 1;
maxIt = 200;
for n = 1:maxIt
    avg = (min + max) / 2;
    res = error(avg, Cd_injector, area_injector, rho, Ptank, Cv_valves, pchamber, rho_h2o);
    if abs((avg-res) / res) < 0.0001
        break;
    end
    if res > avg
        max = avg;
    else
        min = avg;
    end
end
fuel_mdot = res;
end

function md = error(mdot, Cd_injector, area_injector, rho, Ptank, Cv_valves, pchamber, rho_h2o)
    md = Cd_injector * area_injector * sqrt(2 * rho * (Ptank - mdot^2 / (Cv_valves^2 * rho * rho_h2o) - pchamber));
end

== matlab function LR_Traject_Sim/Engine Fluid Sys Model/MATLAB Function ==
  data: temp_kelvin input; specific_enthalpy output
function specific_enthalpy = ox_exit_enthalpy(temp_kelvin)
Trange = 260:1:309;
enthalpies = [137708.762907367,139755.348290231,141812.353420667,143880.113991327,145958.983205259,148049.333206128,150151.556659324,152266.068503765,154393.307897319,156533.740382464,158687.860303283,160856.193510129,163039.300394700,165237.779305935,167452.270406456,169683.460040661,171932.085699494,174198.941684087,176484.885591767,178790.845774488,181117.829953101,183466.935213116,185839.359661369,188236.416092151,190659.548100888,193110.349200556,195590.585650652,198102.223914872,200647.463942151,203228.779846334,205848.970086787,208511.219992905,211219.180533006,213977.068764704,216789.797680403,219663.146607439,222603.988665258,225620.600292982,228723.091839990,231924.021992263,235239.300931658,238689.565367949,242302.362332215,246115.802043553,250185.080407019,254595.158697564,259488.440816707,265136.327556618,272183.585335258,283180.837269871];
%specific_enthalpy = CoolProp.PropsSI('H','T',temp_kelvin,'Q',0,'NITROUSOXIDE');
specific_enthalpy = interp1(Trange, enthalpies, temp_kelvin);
end

== matlab function LR_Traject_Sim/Engine Fluid Sys Model/MATLAB Function1 ==
  data: temp_kelvin input; specific_enthalpy output
function specific_enthalpy = fuel_exit_enthalpy(temp_kelvin)
Trange = 260:1:305;
enthalpies = [204880.334714971,208050.390138587,211240.785849274,214452.161916951,217685.194589443,220940.599479051,224219.135111742,227521.606887504,230848.871498474,234201.841869168,237581.492691768,240988.866647794,244425.081429481,247891.337702528,251388.928187715,254919.248083666,258483.807108706,262084.243508810,265722.340464496,269400.045436794,273119.493127782,276883.032903829,280693.261752904,284553.064139976,288465.660514034,292434.666746810,296464.167506647,300558.807581604,304723.906603823,308965.604712818,313291.049784863,317708.641538307,322228.355103221,326862.178277441,331624.715875657,336534.047351598,341612.982175831,346890.966185823,352407.106622719,358215.236579039,364392.981407536,371059.464607309,378414.264377765,386839.767952767,397265.949220854,413981.931147049];
specific_enthalpy = interp1(Trange, enthalpies, temp_kelvin);
%specific_enthalpy = CoolProp.PropsSI('H','T',temp_kelvin,'Q',0,'ETHANE');
end

== matlab function LR_Traject_Sim/Engine Fluid Sys Model/Combustion chamber model/MATLAB Function3 ==
  data: rho output; T input
function rho = oxdensity(T)
Trange = 260:1:309;
densities = [968.960538442119,964.555134684085,960.106382836984,955.612841552275,951.072988141343,946.485211815440,941.847806201344,937.158961037201,932.416752937820,927.619135100764,922.763925803109,917.848795513144,912.871252410477,907.828626070798,902.718049026446,897.536435858909,892.280459411956,886.946523630991,881.530732431160,876.028853868183,870.436278724405,864.747972418334,858.958418885733,853.061554746050,847.050691635084,840.918424018788,834.656519056104,828.255784082237,821.705905939430,814.995254546292,808.110640555655,801.037013382711,793.757080794342,786.250823859861,778.494870124842,770.461671330684,762.118406390499,753.425489589513,744.334497162176,734.785211936459,724.701285144904,713.983642756544,702.500035071622,690.067600177291,676.421826448870,661.156451382789,643.592930453763,622.445242940298,594.686390337048,548.570585740960];
%rho = CoolProp.PropsSI('D', 'T', T, 'Q', 0, 'NITROUSOXIDE');
rho = interp1(Trange, densities, T);
end

== matlab function LR_Traject_Sim/Engine Fluid Sys Model/Combustion chamber model/MATLAB Function4 ==
  data: rho output; T input
function rho = fueldensity(T)
Trange = 260:1:305;
densities = [429.076168213018,427.062467606728,425.024398601393,422.961031163630,420.871379098400,418.754395003084,416.608964568072,414.433900112595,412.227933273765,409.989706722213,407.717764782997,405.410542818095,403.066355204805,400.683381713451,398.259652045502,395.793028236011,393.281184547713,390.721584382754,388.111453605412,385.447749496481,382.727124336404,379.945882324264,377.099928162542,374.184705142865,371.195119912639,368.125450222587,364.969230755463,361.719110472184,358.366672559390,354.902204669442,351.314402140713,347.589979331509,343.713152495257,339.664938963627,335.422186701185,330.956195950623,326.230701746571,321.198813070513,315.798163820590,309.942813058736,303.508785779834,296.305932390545,288.016278700313,278.032969408980,264.891193367290,241.961491087650];
%rho = CoolProp.PropsSI('D', 'T', T, 'Q', 0, 'ETHANE');
rho = interp1(Trange, densities, T);
end

== matlab function LR_Traject_Sim/MATLAB Function3 ==
  data: CurrentAngle input; drag input; Xaccel output; thrust input; mtotal input; Yaccel output; totalAccel output
function [Xaccel, Yaccel, totalAccel] = AccelerationComponents(CurrentAngle, drag, thrust, mtotal)

%Direction of current velocity vector equals Current Angle
%Thrust and drag are assumed along the axis of the velocity
%Gravity is constant 9.81m/s^2 along the y-axis

%Constants
AccelGravity = -9.81;

AccelDrag = drag/mtotal; %Acceleration caused by drag
AccelThrust = thrust/mtotal; %Acceleration caused by Thrust
AccelRocket = AccelThrust-AccelDrag; %Acceleration of Rocket
Yaccel = AccelRocket * cos(CurrentAngle) + AccelGravity; %Acceleration of Rocket in Y Direction
Xaccel = AccelRocket * sin(CurrentAngle); %Acceleration of rocket in x direction
totalAccel = sqrt(Xaccel^2 + Yaccel^2);

== matlab function LR_Traject_Sim/MATLAB Function4 ==
  data: Xvelo input; CurrentAngle output; Yvelo input; rail_length input; VehicleVelo output; h input; launchangle input
function [CurrentAngle, VehicleVelo]  = CurrentAngle(Xvelo,Yvelo, rail_length, h, launchangle)

%This function's main purpose is to calculate current vehicle angle without
%using two simulink math blocks vs one function block.

%Pretty cool huh?

CurrentAngle = atan(Xvelo/Yvelo);
VehicleVelo = sqrt(Xvelo^2+Yvelo^2);

if h < rail_length
    CurrentAngle = launchangle;
end

== matlab function LR_Traject_Sim/INS Modelling/Total Pressure Transducer/MATLAB Function ==
  data: Pinf input; Ptotal output; rho input; M input
function Ptotal = fcn(Pinf, rho, M)
% Returns the total pressure, selecting an isentropic, or
% Rayleigh formula as appropriate
% Isentropic works just as well as incompressible for our purposes

y = 1.4;

if M > 1
    Ptotal = Pinf * ((((y + 1)^2 * M^2)/(4 * y * M^2 - 2 * (y - 1)))^(y/(y - 1))) * ((1 - y + 2 * y * M^2)/(y + 1));
else
    Ptotal = Pinf * (1 + ((y - 1) * M^2 / 2))^(y / (y - 1));
end
end

== matlab function LR_Traject_Sim/INS Modelling/MATLAB Function1 ==
  data: timestep input; vel input; lastheight input; height output
function height = fcn(timestep, vel, lastheight)

height = lastheight + timestep * vel;
end

== matlab function LR_Traject_Sim/INS Modelling/Predictor ==
  data: timestep input; time input; projected_apogee output; vel input; height input; est_cd input; est_A input; est_mass input; enabled input
function projected_apogee = fcn(timestep, time, vel, height, est_cd, est_A, est_mass, enabled)
if (enabled == 1)
    max_time = 100; %In case something goes wrong it doesn't go into an infinite loop
    
    %cd = 0.433;
    %A = 0.0190106696733447;
    %mass = 32.5516;
    
    cd = est_cd;
    A = est_A;
    mass = est_mass;
    
    while(true)
        lastheight = height;
        time = time + timestep;
        
        p = getStandardPressure(height);
        rho = p/(287.058*(getStandardTemperature(getGeopotential(height/1000))));
        
        accel = -9.81 - ((1/2)*rho*A*cd*vel^2)/mass;
        vel = vel + accel*timestep;
        height = height + vel*timestep;
        
        if(lastheight > height || time > max_time); break; end
    end
end
projected_apogee = height;
end

% stuff below this stolen from wikipedia
function pressure = getStandardPressure( altitude)

altitude = altitude / 1000.0;
geopot_height = getGeopotential(altitude);

t = getStandardTemperature(geopot_height);

pressure = 0;
if (geopot_height <= 11)
    pressure = 101325 * (288.15 / t)^( -5.255877);
elseif (geopot_height <= 20)
    pressure = 22632.06 * exp(-0.1577 * (geopot_height - 11));
elseif (geopot_height <= 32)
    pressure = 5474.889 * (216.65 / t)^( 34.16319);
elseif (geopot_height <= 47)
    pressure = 868.0187 * (228.65 / t)^( 12.2011);
elseif (geopot_height <= 51)
    pressure = 110.9063 * exp(-0.1262 * (geopot_height - 47));
elseif (geopot_height <= 71)
    pressure = 66.93887 * (270.65 / t)^( -12.2011);
elseif (geopot_height <= 84.85)
    pressure = 3.956420 * (214.65 / t)^( -17.0816);
end

end

function temperature = getStandardTemperature(geopot_height)

temperature = 273.15;
if (geopot_height <= 11)
    temperature = 288.15 - (6.5 * geopot_height);
elseif (geopot_height <= 20)
    temperature = 216.65;
elseif (geopot_height <= 32)
    temperature = 196.65 + geopot_height;
elseif (geopot_height <= 47)
    temperature = 228.65 + 2.8 * (geopot_height - 32);
elseif (geopot_height <= 51)
    temperature = 270.65;
elseif (geopot_height <= 71)
    temperature = 270.65 - 2.8 * (geopot_height - 51);
elseif (geopot_height <= 84.85)
    temperature = 214.65 - 2 * (geopot_height - 71); 
end

end

function geopot = getGeopotential(altitude_km)

EARTH_RADIUS = 6356.766;

geopot = EARTH_RADIUS * altitude_km / (EARTH_RADIUS + altitude_km);
end
